simulink model "PV4kW"  (R2024a)
settings: Solver=VariableStepAuto  StartTime=0.0  StopTime=1  RelTol=1e-3
libraries: spsDiodeLib x9, spsPVArrayLib x9, spsControlledVoltageSourceLib x1, spsCurrentMeasurementLib x1, simulink x1, spsVoltageMeasurementLib x1, sps_lib x1
settings Model: Creator=Rahuldev  LastModifiedBy=Rahuldev

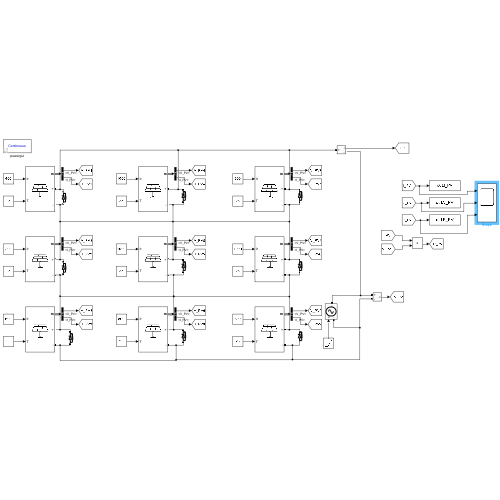
[thumbnail: Simulink's stored preview of the top-level diagram]
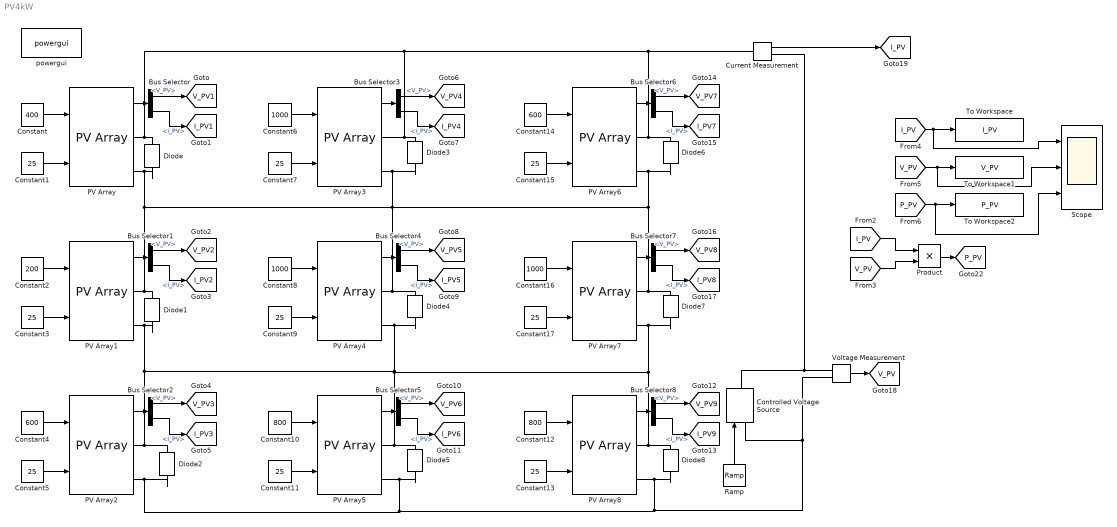
== system PV4kW ==
  Bus Selector{,1..8} (9 alike) : BusSelector  OutputSignals=V_PV,I_PV
  Constant : Constant  Value=400
  Constant{1,3,5,7,9,11,13,15,17} (9 alike) : Constant  Value=25
  Constant10 : Constant  Value=800
  Constant12 : Constant  Value=800
  Constant14 : Constant  Value=600
  Constant16 : Constant  Value=1000
  Constant2 : Constant  Value=200
  Constant4 : Constant  Value=600
  Constant6 : Constant  Value=1000
  Constant8 : Constant  Value=1000
  Controlled Voltage Source : spsControlledVoltageSourceLib/Controlled Voltage Source  Initialize=on  Source_Type=DC  Amplitude=0  Phase=0  Frequency=0  Measurements=None
  Current Measurement : spsCurrentMeasurementLib/Current Measurement  PhasorSimulation=off  OutputType=Complex  PSBequivalent=0
  Diode{,1..8} (9 alike) : spsDiodeLib/Diode  Ron=0.001  Lon=0  Vf=0.8  IC=0  UseSnubber=0  Rs=500  Cs=250e-9  Measurements=off
  PV Array{,1..8} (9 alike) : spsPVArrayLib/PV Array  Npar=1  Nser=1  PlotType=array @ 25 deg.C & specified irradiances  S_vec="[ 1000  800  600  400  200 ]"  Temp_C_vec="[ 45 25  ]"  ModuleName=User-defined  PlotWhenSelected=off  Pm=540.474  Ncell=144  Voc=49.32  Isc=13.71  Vm=41.80  Im=12.93  beta_Voc_pc=-0.28  alpha_Isc_pc=0.048  beta_Voc=-0.1381  alpha_Isc=0.0065808  IL=13.7275  I0=1.9489e-11  nI=0.48903  Rsh=175.1393  Rs=0.14047  RobustModel=off  RobustCellTemperature=313.3991  BAL=on  Tc=1e-6  Tfilter=5e-5
  Product : Product
  Ramp : simulink/Sources/Ramp  slope=145.77  start=0  InitialOutput=0
  Scope : Scope  NumInputPorts=3
  To Workspace : ToWorkspace  VariableName=I_PV  SaveFormat=Structure With Time  SampleTime=-1
  To Workspace1 : ToWorkspace  VariableName=V_PV  SaveFormat=Structure With Time  SampleTime=-1
  To Workspace2 : ToWorkspace  VariableName=P_PV  SaveFormat=Structure With Time  SampleTime=-1
  Voltage Measurement : spsVoltageMeasurementLib/Voltage Measurement  PhasorSimulation=off  OutputType=Complex  PSBequivalent=0
  powergui : sps_lib/powergui  Priority=1  SimulationMode=Continuous  SampleTime=50e-6  frequency=60  Iterations=50  frequencyindice=0  Pbase=100e6  ErrMax=1e-4  UnitsV=kV  UnitsW=MW  buscounter=0  FunctionMessages=off  echomessages=off  EnableUseOfTLC=off  CurrentSourceSwitches=off  DisableSnubberDevices=off  DisableRonSwitches=off  DisableVfSwitches=off  DisplayEquations=off  AutomaticDiscreteSolvers=off  SolverType=Tustin/Backward Euler (TBE)  Interpol=off  ExternalGateDelay=off  methode=off  Ts=100  x0status=blocks  SPID=on  SwTol=0  HookPort=off  NonlinearTolerance=1e-4  nMaxIteration=100  ContinueOnMaxIteration=off  RestoreLinks=warning  ResistiveCurrentMeasurement=off  Frange=[0:2:500]  Ylog=off  Xlog=on  ShowGrid=off  save=off  variable=ZData  structure=0  ZoomFFT=off  StartTime=0.0  cycles=1  DisplayStyle=1  fundamental=60  FreqAxis=off  MaxFrequency=1000  frequencyindicesteady=1  RmsSteady=1  display=off
  tag scope: I_PV1=global, I_PV2=global, I_PV3=global, I_PV4=global, I_PV5=global, I_PV6=global, I_PV7=global, I_PV8=global, I_PV9=global, I_PV=global, P_PV=global, V_PV1=global, V_PV2=global, V_PV3=global, V_PV4=global, V_PV5=global, V_PV6=global, V_PV7=global, V_PV8=global, V_PV9=global, V_PV=global
  wires:
  Constant4/1 -> PV Array2/1
  Constant5/1 -> PV Array2/2
  Bus Selector4/2 -> [I_PV5]  "<I_PV>"
  Bus Selector3/1 -> [V_PV4]  "<V_PV>"
  PV Array3/1 -> Bus Selector3/1
  Constant7/1 -> PV Array3/2
  Constant8/1 -> PV Array4/1
  Constant10/1 -> PV Array5/1
  Constant9/1 -> PV Array4/2
  Bus Selector5/2 -> [I_PV6]  "<I_PV>"
  Bus Selector/1 -> [V_PV1]  "<V_PV>"
  PV Array1/1 -> Bus Selector1/1
  Bus Selector1/1 -> [V_PV2]  "<V_PV>"
  Constant3/1 -> PV Array1/2
  PV Array2/1 -> Bus Selector2/1
  Bus Selector/2 -> [I_PV1]  "<I_PV>"
  PV Array/1 -> Bus Selector/1
  Constant1/1 -> PV Array/2
  Bus Selector8/1 -> [V_PV9]  "<V_PV>"
  PV Array8/1 -> Bus Selector8/1
  Constant12/1 -> PV Array8/1
  Constant11/1 -> PV Array5/2
  Constant17/1 -> PV Array7/2
  Bus Selector6/1 -> [V_PV7]  "<V_PV>"
  Bus Selector7/1 -> [V_PV8]  "<V_PV>"
  Bus Selector2/2 -> [I_PV3]  "<I_PV>"
  Constant15/1 -> PV Array6/2
  Constant14/1 -> PV Array6/1
  Bus Selector5/1 -> [V_PV6]  "<V_PV>"
  PV Array4/1 -> Bus Selector4/1
  Current Measurement/1 -> [I_PV]
  Bus Selector7/2 -> [I_PV8]  "<I_PV>"
  Bus Selector2/1 -> [V_PV3]  "<V_PV>"
  Bus Selector6/2 -> [I_PV7]  "<I_PV>"
  Voltage Measurement/1 -> [V_PV]
  Constant2/1 -> PV Array1/1
  Constant/1 -> PV Array/1
  Constant13/1 -> PV Array8/2
  PV Array5/1 -> Bus Selector5/1
  Bus Selector4/1 -> [V_PV5]  "<V_PV>"
  Constant16/1 -> PV Array7/1
  Constant6/1 -> PV Array3/1
  Bus Selector8/2 -> [I_PV9]  "<I_PV>"
  PV Array6/1 -> Bus Selector6/1
  PV Array7/1 -> Bus Selector7/1
  Bus Selector1/2 -> [I_PV2]  "<I_PV>"
  Bus Selector3/2 -> [I_PV4]  "<I_PV>"
  Product/1 -> [P_PV]
  [I_PV] -> Scope/1, To Workspace/1
  [V_PV] -> Scope/2, To Workspace1/1
  [I_PV] -> Product/1
  [V_PV] -> Product/2
  [P_PV] -> Scope/3, To Workspace2/1
  Ramp/1 -> Controlled Voltage Source/1
  connections:
  PV Array1/RConn1 -- Diode/LConn1 -- PV Array/RConn2 -- Diode6/LConn1 -- PV Array6/RConn2 -- Diode7/RConn1 -- PV Array7/RConn1 -- Diode3/LConn1 -- PV Array3/RConn2 -- Diode4/RConn1 -- PV Array4/RConn1 -- Diode1/RConn1
  Current Measurement/LConn1 -- PV Array3/RConn1 -- Diode3/RConn1 -- PV Array/RConn1 -- Diode/RConn1 -- Diode6/RConn1 -- PV Array6/RConn1
  Diode1/LConn1 -- PV Array1/RConn2 -- PV Array2/RConn1 -- Diode2/RConn1 -- PV Array5/RConn1 -- Diode5/RConn1 -- Diode7/LConn1 -- PV Array7/RConn2 -- Diode8/RConn1 -- PV Array8/RConn1 -- PV Array4/RConn2 -- Diode4/LConn1
  Diode2/LConn1 -- PV Array2/RConn2 -- Diode5/LConn1 -- PV Array5/RConn2 -- Voltage Measurement/LConn2 -- Controlled Voltage Source/LConn1 -- Diode8/LConn1 -- PV Array8/RConn2
  Current Measurement/RConn1 -- Controlled Voltage Source/RConn1 -- Voltage Measurement/LConn1
